simulink model "matlab_simulink"  (R2023a)
settings: Solver=VariableStepAuto  StartTime=0.0  StopTime=5  RelTol=1e-3
InitFcn:
  | u = udpport;
  | writeline(u,"M;2B8:i;574:i;", "127.0.0.1", 27015)
  | writeline(u,"C;310A:c;089A:s;", "127.0.0.1", 27015)
undefined symbols (not defined in the file): f
libraries: instrumentlib x2
settings Model: Creator=asd  LastModifiedBy=asd

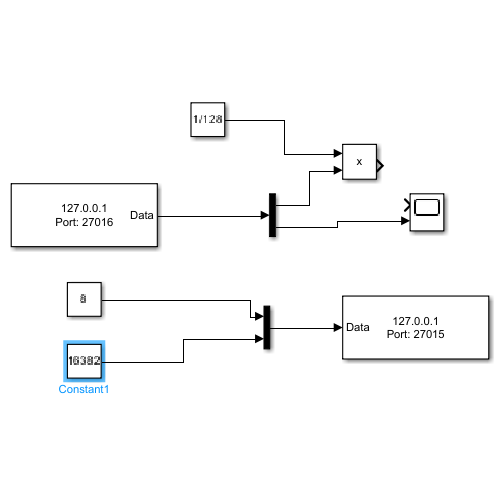
[thumbnail: Simulink's stored preview of the top-level diagram]
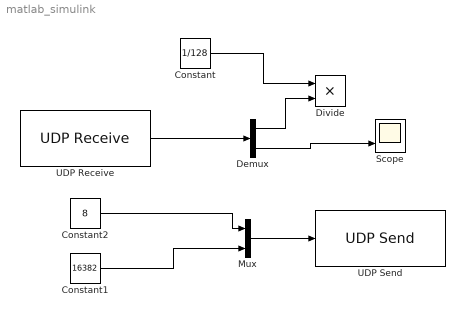
== system matlab_simulink ==
  Constant : Constant  Value=1/128
  Constant1 : Constant  Value=16382
  Constant2 : Constant  Value=8
  Demux : Demux  Outputs=2
  Divide : Product
  Mux : Mux  Inputs=2
  Scope : Scope  NumInputPorts=2
  UDP Receive : instrumentlib/UDP Receive  LocalAddress=127.0.0.1  LocalPort=27016  EnablePortSharing=off  Host=127.0.0.1  Port=27015  GetLatestData=off  DataSize=[2, 1]  DataType=double  ASCIIFormatting=%f,  Terminator=LF  CustomTerminator=10  ByteOrder=big-endian  EnableBlockingMode=on  Timeout=10  SampleTime=0.1  SimulateUsing=Interpreted execution
  UDP Send : instrumentlib/UDP Send  Host=127.0.0.1  Port=27015  LocalAddress=0.0.0.0  LocalPort=-1  EnablePortSharing=off  OutputDatagramPacketSize=512  ByteOrder=big-endian  EnableBlockingMode=on  SimulateUsing=Interpreted execution
  wires:
  UDP Receive/1 -> Demux/1
  Demux/1 -> Divide/2
  Demux/2 -> Scope/2
  Constant/1 -> Divide/1
  Constant2/1 -> Mux/1
  Constant1/1 -> Mux/2
  Mux/1 -> UDP Send/1
